simulink model "UAVIntegratedNavigationSystem"  (R2020b)
settings: Solver=FixedStepAuto  StartTime=0.0  StopTime=TFinal  FixedStep=IMUtime  RelTol=1e-3
values from neighbouring files (symbols this model uses):
  AIONtime = 1    [ModelSettings.m]
  BiasAccel = 9.81E-4    (= 0.000981)    [ModelSettings.m]
  BiasGyro = 2.424068405548E-4    (= 0.000242406840555)    [ModelSettings.m]
  CorrTimeOrientationGNSS = 1    [ModelSettings.m]
  CorrTimePositionGNSS = 1    [ModelSettings.m]
  CorrTimeVelocityGNSS = 1    [ModelSettings.m]
  delay = 1.5    [ModelSettings.m]
  e = 0.081819106    [ModelSettings.m]
  g0 = 9.780327    [ModelSettings.m]
  GNSStime = 0.2    [ModelSettings.m]
  H0 = 0.1    [ModelSettings.m]
  IMUtime = 0.01    [ModelSettings.m]
  indUAV = 2    [ModelSettings.m]
  LambdaInit = 0.6555    [ModelSettings.m]
  mass = 0.7    [ModelSettings.m]
  N = 100    [ModelSettings.m]
  PhiInit = 0.968    [ModelSettings.m]
  PitchDown = -PitchUp    (= -0.1)    [ModelSettings.m]
  PitchUp = 0.1    [ModelSettings.m]
  Ra = 6378.245    [ModelSettings.m]
  RollDown = -RollUp    (= -0.1)    [ModelSettings.m]
  RollUp = 0.1    [ModelSettings.m]
  SigmaAccel = 9.81E-4    (= 0.000981)    [ModelSettings.m]
  SigmaAION = 30    [ModelSettings.m]
  SigmaAltitudeGNSS = 3    [ModelSettings.m]
  SigmaGyro = 2.666475246102E-6    (= 2.6664752461e-06)    [ModelSettings.m]
  SigmaLaser = 5    [ModelSettings.m]
  SigmaOrientationGNSS = 0.00349    [ModelSettings.m]
  SigmaPositionGNSS = 1.5    [ModelSettings.m]
  SigmaVelocityGNSS = 0.03    [ModelSettings.m]
  SigmaVelocityUpGNSS = 0.03    [ModelSettings.m]
  U1down = 0    [ModelSettings.m]
  U1up = 4 * ForceCoeff * OmegaMax^2    (= 9.9858124)    [ModelSettings.m]
  U2down = -U2up    (= -2.4964531)    [ModelSettings.m]
  U2up = ForceCoeff * OmegaMax^2    (= 2.4964531)    [ModelSettings.m]
  U3down = -U3up    (= -2.4964531)    [ModelSettings.m]
  U3up = ForceCoeff * OmegaMax^2    (= 2.4964531)    [ModelSettings.m]
  U4down = -U4up    (= -0.2494604)    [ModelSettings.m]
  U4up = 2 * DragCoeff * OmegaMax^2    (= 0.2494604)    [ModelSettings.m]
  WEarth = 7.2921158553E-5    (= 7.2921158553e-05)    [ModelSettings.m]
undefined symbols (not defined in the file or in its folder): deg, Newton, rad, Raphson, s
libraries: simulink x11, sharedtransform x7, pid_lib x6, aerolibconvert2 x4, sharedutil x4
(part 2 of 5)

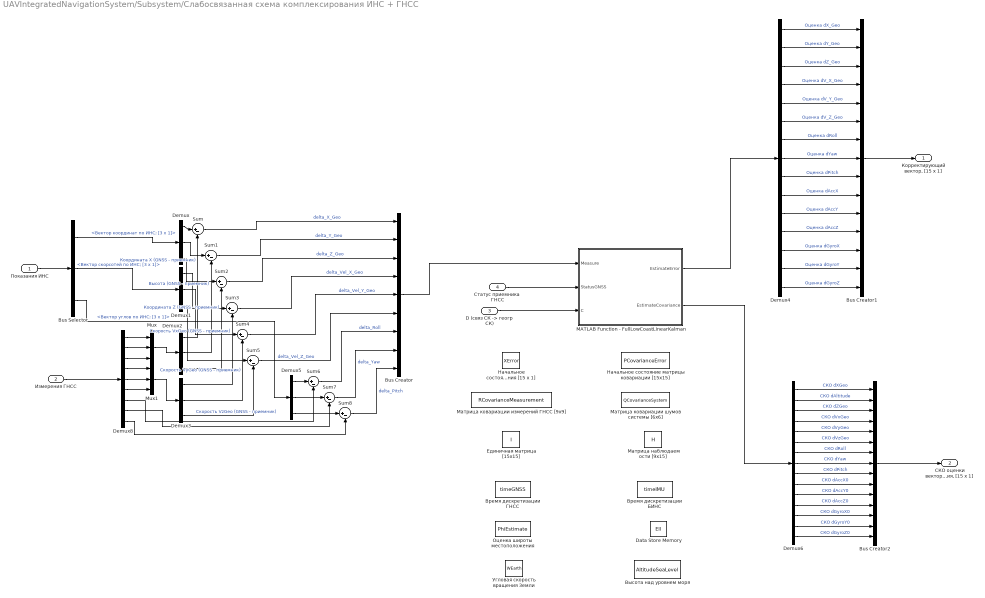
== system UAVIntegratedNavigationSystem/Subsystem/Слабосвязанная схема комплексирования ИНС + ГНСС ==
  Показания ИНС : Inport
  Измерения ГНСС : Inport  Port=2  SampleTime=0.1
  "D (связ СК -> геогр СК)" : Inport  Port=3
  Статус приемника  ГНСС : Inport  Port=4
  Bus Creator : BusCreator  Inputs=9
  Bus Creator1 : BusCreator  Inputs=15
  Bus Creator2 : BusCreator  Inputs=15
  Bus Selector : BusSelector  OutputSignals=Вектор координат по ИНС; [3 x 1],Вектор скорсотей по ИНС; [3 x 1],Вектор углов по ИНС; [3 x 1]
  Data Store Memory : DataStoreMemory  DataStoreName=Ell  ReadBeforeWriteMsg=warning  WriteAfterWriteMsg=warning  WriteAfterReadMsg=warning  InitialValue=[Ra;e]  ShowAdditionalParam=off  OutDataTypeStr=double
  Demux{,1..3,5} (5 alike) : Demux  Outputs=3
  Demux4 : Demux  Outputs=15
  Demux6 : Demux  Outputs=15
  Demux8 : Demux  Outputs=9
  MATLAB Function - FullLowCoastLinearKalman : MATLAB Function  TreatAsAtomicUnit=on
  Mux : Mux  Inputs=3
  Mux1 : Mux  Inputs=3
  Sum{,1..8} (9 alike) : Sum  Inputs=|+-
  Время дискретизации БИНС : DataStoreMemory  DataStoreName=timeIMU  ReadBeforeWriteMsg=warning  WriteAfterWriteMsg=warning  WriteAfterReadMsg=warning  InitialValue=1E-2  ShowAdditionalParam=off  OutDataTypeStr=double
  Время дискретизации ГНСС : DataStoreMemory  DataStoreName=timeGNSS  ReadBeforeWriteMsg=warning  WriteAfterWriteMsg=warning  WriteAfterReadMsg=warning  InitialValue=GNSStime  ShowAdditionalParam=off  OutDataTypeStr=double
  Высота над уровнем моря : DataStoreMemory  DataStoreName=AltitudeSeaLevel  ReadBeforeWriteMsg=warning  WriteAfterWriteMsg=warning  WriteAfterReadMsg=warning  InitialValue=H0  ShowAdditionalParam=off  OutDataTypeStr=double
  Единичная матрица [15x15] : DataStoreMemory  DataStoreName=I  ReadBeforeWriteMsg=warning  WriteAfterWriteMsg=warning  WriteAfterReadMsg=warning  InitialValue=eye(15)  ShowAdditionalParam=off  OutDataTypeStr=double
  Матрица ковариации измерений ГНСС [9x9] : DataStoreMemory  DataStoreName=RCovarianceMeasurement  ReadBeforeWriteMsg=warning  WriteAfterWriteMsg=warning  WriteAfterReadMsg=warning  InitialValue="diag([ (0.1 * SigmaPositionGNSS)^2 (0.1 * SigmaAltitudeGNSS)^2 (0.1 * SigmaPositionGNSS)^2  (1*SigmaVelocityGNSS)^2  (1*SigmaVelocityUpGNSS)^2 (1*SigmaVelocityGNSS)^2 (0.001*SigmaOrientationGNSS)^2 (0.001*SigmaOrientationGNSS)^2 (0.001*SigmaOrientationGNSS)^2])"  ShowAdditionalParam=off  OutDataTypeStr=double
  Матрица ковариации шумов системы [6x6] : DataStoreMemory  DataStoreName=QCovarianceSystem  ReadBeforeWriteMsg=warning  WriteAfterWriteMsg=warning  WriteAfterReadMsg=warning  InitialValue=diag([SigmaAccel^2 SigmaAccel^2 SigmaAccel^2 SigmaGyro^2 SigmaGyro^2 SigmaGyro^2])  ShowAdditionalParam=off  OutDataTypeStr=double
  Матрица наблюдаемости [9x15] : DataStoreMemory  DataStoreName=H  ReadBeforeWriteMsg=warning  WriteAfterWriteMsg=warning  WriteAfterReadMsg=warning  InitialValue=[1 0 0 0 0 0 0 0 0 0 0 0 0 0 0;0 1 0 0 0 0 0 0 0 0 0 0 0 0 0; 0 0 1 0 0 0 0 0 0 0 0 0 0 0 0; 0 0 0 1 0 0 0 0 0 0 0 0 0 0 0; 0 0 0 0 1 0 0 0 0 0 0 0 0 0 0; 0 0 0 0 0 1 0 0 0 0 0 0 0 0 0; 0 0 0 0 0 0 1 0 0 0 0 0 0 0 0; 0 0 0 0 0 0 0 1 0 0 0 0 0 0 0; 0 0 0 0 0 0 0 0 1 0 0 0 0 0 0]  ShowAdditionalParam=off  OutDataTypeStr=double
  Начальное состояние вектора - состояния [15 x 1] : DataStoreMemory  DataStoreName=XError  ReadBeforeWriteMsg=warning  WriteAfterWriteMsg=warning  WriteAfterReadMsg=warning  InitialValue=[0;0;0;0;0;0;0;0;0;0;0;0;0;0;0]  ShowAdditionalParam=off  OutDataTypeStr=double
  Начальное состояние матрицы ковариации [15x15] : DataStoreMemory  DataStoreName=PCovarianceError  ReadBeforeWriteMsg=warning  WriteAfterWriteMsg=warning  WriteAfterReadMsg=warning  InitialValue=diag([10 10 10 2 2 2 1e-1 1e-1 1e-1 1e-3 1e-3 1e-3 1e-3 1e-3 1e-3])  ShowAdditionalParam=off  OutDataTypeStr=double
  Оценка широты местоположения : DataStoreMemory  DataStoreName=PhiEstimate  ReadBeforeWriteMsg=warning  WriteAfterWriteMsg=warning  WriteAfterReadMsg=warning  InitialValue=PhiInit  ShowAdditionalParam=off  OutDataTypeStr=double
  Угловая скорость вращения Земли : DataStoreMemory  DataStoreName=WEarth  ReadBeforeWriteMsg=warning  WriteAfterWriteMsg=warning  WriteAfterReadMsg=warning  InitialValue=WEarth  ShowAdditionalParam=off  OutDataTypeStr=double
  "Корректирующий вектор, [15 x 1]" : Outport
  "СКО оценки вектора состояния, [15 x 1]" : Outport  Port=2
  wires:
  Показания ИНС/1 -> Bus Selector/1
  Sum/1 -> Bus Creator/1  "delta_X_Geo"
  Sum1/1 -> Bus Creator/2  "delta_Y_Geo"
  Sum2/1 -> Bus Creator/3  "delta_Z_Geo"
  Sum3/1 -> Bus Creator/4  "delta_Vel_X_Geo"
  Sum4/1 -> Bus Creator/5  "delta_Vel_Y_Geo"
  Demux3/2 -> Sum4/2  "Скорость VyGeo (GNSS - приемник)"
  Sum5/1 -> Bus Creator/6  "delta_Vel_Z_Geo"
  Demux3/3 -> Sum5/2  "Скорость VzGeo (GNSS - приемник)"
  Bus Selector/1 -> Demux/1  "<Вектор координат по ИНС; [3 x 1]>"
  Bus Selector/2 -> Demux1/1  "<Вектор скорсотей по ИНС; [3 x 1]>"
  Demux8/1 -> Mux/1
  Demux8/2 -> Mux/2
  Demux8/3 -> Mux/3
  Mux/1 -> Demux2/1
  Demux8/4 -> Mux1/1
  Demux8/5 -> Mux1/2
  Demux8/6 -> Mux1/3
  Mux1/1 -> Demux3/1
  Demux6/1 -> Bus Creator2/1  "СКО dXGeo"
  Demux6/2 -> Bus Creator2/2  "СКО dAltitude"
  Demux6/3 -> Bus Creator2/3  "СКО dZGeo"
  Demux6/4 -> Bus Creator2/4  "СКО dVxGeo"
  Demux6/5 -> Bus Creator2/5  "СКО dVyGeo"
  Demux6/6 -> Bus Creator2/6  "СКО dVzGeo"
  Demux/1 -> Sum/1
  Demux2/1 -> Sum/2  "Координата X (GNSS - приемник)"
  Demux/2 -> Sum1/1
  Demux2/2 -> Sum1/2  "Высота (GNSS - приемник)"
  Demux2/3 -> Sum2/2  "Координата Z (GNSS - приемник)"
  Demux/3 -> Sum2/1
  Demux1/1 -> Sum3/1
  Demux3/1 -> Sum3/2  "Скорость VxGeo (GNSS - приемник)"
  Demux1/3 -> Sum5/1
  Demux1/2 -> Sum4/1
  Demux4/1 -> Bus Creator1/1  "Оценка dX_Geo"
  Demux4/2 -> Bus Creator1/2  "Оценка dY_Geo"
  Demux4/3 -> Bus Creator1/3  "Оценка dZ_Geo"
  Demux4/4 -> Bus Creator1/4  "Оценка dV_X_Geo"
  Demux4/5 -> Bus Creator1/5  "Оценка dV_Y_Geo"
  Demux4/6 -> Bus Creator1/6  "Оценка dV_Z_Geo"
  Demux4/7 -> Bus Creator1/7  "Оценка dRoll"
  Demux4/8 -> Bus Creator1/8  "Оценка dYaw"
  Demux4/9 -> Bus Creator1/9  "Оценка dPitch"
  Demux6/7 -> Bus Creator2/7  "СКО dRoll"
  Demux6/8 -> Bus Creator2/8  "СКО dYaw"
  Demux6/9 -> Bus Creator2/9  "СКО dPitch"
  Bus Creator2/1 -> "СКО оценки вектора состояния, [15 x 1]"/1
  "D (связ СК -> геогр СК)"/1 -> MATLAB Function - FullLowCoastLinearKalman/3(C)
  Bus Selector/3 -> Demux5/1  "<Вектор углов по ИНС; [3 x 1]>"
  Demux5/1 -> Sum6/1
  Demux8/7 -> Sum6/2
  Sum6/1 -> Bus Creator/7  "delta_Roll"
  Demux5/2 -> Sum7/1
  Sum7/1 -> Bus Creator/8  "delta_Yaw"
  Demux8/8 -> Sum7/2
  Demux5/3 -> Sum8/1
  Sum8/1 -> Bus Creator/9  "delta_Pitch"
  Demux8/9 -> Sum8/2
  Bus Creator/1 -> MATLAB Function - FullLowCoastLinearKalman/1(Measure)
  Demux6/10 -> Bus Creator2/10  "СКО dAccX0"
  Demux6/11 -> Bus Creator2/11  "СКО dAccY0"
  Demux6/12 -> Bus Creator2/12  "СКО dAccZ0"
  Demux6/13 -> Bus Creator2/13  "СКО dGyroX0"
  Demux6/14 -> Bus Creator2/14  "СКО dGyroY0"
  Demux6/15 -> Bus Creator2/15  "СКО dGyroZ0"
  Demux4/10 -> Bus Creator1/10  "Оценка dAccX"
  Demux4/11 -> Bus Creator1/11  "Оценка dAccY"
  Demux4/12 -> Bus Creator1/12  "Оценка dAccZ"
  Demux4/13 -> Bus Creator1/13  "Оценка dGyroX"
  Demux4/14 -> Bus Creator1/14  "Оценка dGyroY"
  Demux4/15 -> Bus Creator1/15  "Оценка dGyroZ"
  MATLAB Function - FullLowCoastLinearKalman/2(EstimateCovariance) -> Demux6/1
  Измерения ГНСС/1 -> Demux8/1
  Статус приемника  ГНСС/1 -> MATLAB Function - FullLowCoastLinearKalman/2(StatusGNSS)
  MATLAB Function - FullLowCoastLinearKalman/1(EstimateError) -> Demux4/1
  Bus Creator1/1 -> "Корректирующий вектор, [15 x 1]"/1

== system UAVIntegratedNavigationSystem/Subsystem1/Функционирование АИОН ==
  КОИ : Inport
  Измерения АИОН : Inport  Port=2
  Bus Creator : BusCreator  Inputs=3
  Data Store Memory : DataStoreMemory  DataStoreName=sum  ReadBeforeWriteMsg=warning  WriteAfterWriteMsg=warning  WriteAfterReadMsg=warning  ShowAdditionalParam=off  OutDataTypeStr=double
  Demux : Demux  Outputs=3
  If Action Subsystem1 : Subsystem  TreatAsAtomicUnit=on
  If Action Subsystem3 : Subsystem  TreatAsAtomicUnit=on
  If Action Subsystem4 : Subsystem  TreatAsAtomicUnit=on
  If Action Subsystem5 : Subsystem  TreatAsAtomicUnit=on
  MATLAB Function : MATLAB Function  TreatAsAtomicUnit=on
  Merge : Merge
  Merge1 : Merge
  Rate Transition : RateTransition  OutPortSampleTime=AIONtime
  Моменты получения информации с АИОН : DiscretePulseGenerator  PulseType=Time based  Period=AIONtime  PulseWidth=10  PhaseDelay=GNSStime
  Отказ  АИОН : If  IfExpression=u1 == 2
  Пропадание имзерений АИОН : If  IfExpression=u1 == -1
  Измерения АИОН (выход) : Outport
  Статус АИОН (-1/0 / 1) : Outport  Port=2
  Количество отсчетов после проадания сигнала АИОН : Outport  Port=3
  wires:
  If Action Subsystem1/1(Out1) -> Merge/1
  If Action Subsystem3/1(Out1) -> Merge/2
  Пропадание имзерений АИОН/1 -> If Action Subsystem4/Action
  Измерения АИОН/1 -> If Action Subsystem5/1(In1)
  Пропадание имзерений АИОН/2 -> If Action Subsystem5/Action
  If Action Subsystem4/1(Out1) -> Merge1/1
  If Action Subsystem5/1(Out1) -> Merge1/2
  Merge1/1 -> Demux/1
  КОИ/1 -> Отказ  АИОН/1
  Отказ  АИОН/1 -> If Action Subsystem1/Action
  Отказ  АИОН/2 -> If Action Subsystem3/Action
  Моменты получения информации с АИОН/1 -> If Action Subsystem1/1(In1)
  Demux/1 -> Bus Creator/1  "X_Geo_AION"
  Demux/2 -> Bus Creator/2  "Altitude_AION"
  Demux/3 -> Bus Creator/3  "Z_Geo_AION"
  Bus Creator/1 -> Измерения АИОН (выход)/1
  Merge/1 -> Статус АИОН (-1/0 / 1)/1, MATLAB Function/1(AIONStatus), Пропадание имзерений АИОН/1
  MATLAB Function/1(y) -> Rate Transition/1
  Rate Transition/1 -> Количество отсчетов после проадания сигнала АИОН/1

== system UAVIntegratedNavigationSystem/Subsystem1/Функционирование приемника ГНСС ==
  КОИ : Inport
  Измерения приемника ГНСС : Inport  Port=2
  Bus Creator : BusCreator  Inputs=3
  Data Store Memory : DataStoreMemory  DataStoreName=sum  ReadBeforeWriteMsg=warning  WriteAfterWriteMsg=warning  WriteAfterReadMsg=warning  ShowAdditionalParam=off  OutDataTypeStr=double
  Demux : Demux  Outputs=9
  If Action Subsystem1 : Subsystem  TreatAsAtomicUnit=on
  If Action Subsystem3 : Subsystem  TreatAsAtomicUnit=on
  If Action Subsystem4 : Subsystem  TreatAsAtomicUnit=on
  If Action Subsystem5 : Subsystem  TreatAsAtomicUnit=on
  MATLAB Function : MATLAB Function  TreatAsAtomicUnit=on
  Merge : Merge
  Merge1 : Merge
  Mux : Mux  Inputs=3
  Mux1 : Mux  Inputs=3
  Mux2 : Mux  Inputs=3
  Rate Transition : RateTransition  OutPortSampleTime=GNSStime
  Моменты получения информации с ГНСС : DiscretePulseGenerator  PulseType=Time based  Period=GNSStime  PulseWidth=10  PhaseDelay=GNSStime
  Отказ  приемника ГНСС : If  IfExpression=u1 == 1
  Пропадание измерений приемника ГНСС : If  IfExpression=u1 == -1
  Измерения приемника ГНСС (выход) : Outport
  Статус приемника (-1/0 / 1) : Outport  Port=2
  Количество отсчетов после проадания сигнала ГНСС : Outport  Port=3
  wires:
  If Action Subsystem1/1(Out1) -> Merge/1
  If Action Subsystem3/1(Out1) -> Merge/2
  Пропадание измерений приемника ГНСС/1 -> If Action Subsystem4/Action
  Измерения приемника ГНСС/1 -> If Action Subsystem5/1(In1)
  Пропадание измерений приемника ГНСС/2 -> If Action Subsystem5/Action
  If Action Subsystem4/1(Out1) -> Merge1/1
  If Action Subsystem5/1(Out1) -> Merge1/2
  КОИ/1 -> Отказ  приемника ГНСС/1
  Отказ  приемника ГНСС/1 -> If Action Subsystem1/Action
  Отказ  приемника ГНСС/2 -> If Action Subsystem3/Action
  Merge/1 -> Статус приемника (-1/0 / 1)/1, Пропадание измерений приемника ГНСС/1, MATLAB Function/1(GNSSStatus)
  Моменты получения информации с ГНСС/1 -> If Action Subsystem1/1(In1)
  Merge1/1 -> Demux/1
  Demux/1 -> Mux/1
  Demux/2 -> Mux/2
  Demux/3 -> Mux/3
  Mux/1 -> Bus Creator/1  "Вектор координат по ГНСС; [3 x 1]"
  Demux/4 -> Mux1/1
  Demux/5 -> Mux1/2
  Demux/6 -> Mux1/3
  Mux1/1 -> Bus Creator/2  "Вектор скоростей по ГНСС; [3 x 1]"
  Bus Creator/1 -> Измерения приемника ГНСС (выход)/1
  Demux/8 -> Mux2/2
  Demux/9 -> Mux2/3
  Demux/7 -> Mux2/1
  Mux2/1 -> Bus Creator/3  "Вектор углов по ГНСС; [3 x 1]"
  MATLAB Function/1(y) -> Rate Transition/1
  Rate Transition/1 -> Количество отсчетов после проадания сигнала ГНСС/1

== system UAVIntegratedNavigationSystem/Алгоритм ИНС /Алгоритм Навигации ==
  Показания акселерометров (геогр СК) : Inport
  "Север(0), Восток(0)" : Inport  Port=2
  Demux : Demux  Outputs=3
  Demux1 : Demux
  Mux : Mux  Inputs=3
  Mux1 : Mux  Inputs=2
  Координаты БПЛА (Географ. СК) : Subsystem
  Радиус - вектор точки местоположения Ц.М. БПЛА (phi) : Subsystem
  Скорости БПЛА (Географ. СК) : Subsystem
  Угловая скорость вращения трехгранника : Subsystem
  "Координаты, скорости БЛА" : Outport
  OmegaG : Outport  Port=2
  Широта местоположения БЛА : Outport  Port=3
  "Радиусы кривизны земного эллипсоида, м" : Outport  Port=4
  wires:
  Demux/1 -> Скорости БПЛА (Географ. СК)/1(AccX)  "AccX"
  Demux/2 -> Скорости БПЛА (Географ. СК)/2(AccY)  "AccY"
  Demux/3 -> Скорости БПЛА (Географ. СК)/3(AccZ)  "AccZ"
  Показания акселерометров (геогр СК)/1 -> Demux/1
  Координаты БПЛА (Географ. СК)/1("Coord, phi") -> Demux1/1
  Demux1/4 -> Угловая скорость вращения трехгранника/3(phi), Скорости БПЛА (Географ. СК)/5(phi), Радиус - вектор точки местоположения Ц.М. БПЛА (phi)/1(Phi), Широта местоположения БЛА/1
  Радиус - вектор точки местоположения Ц.М. БПЛА (phi)/1("R, м") -> Скорости БПЛА (Географ. СК)/4(R), Угловая скорость вращения трехгранника/2(R), Координаты БПЛА (Географ. СК)/2(R), "Радиусы кривизны земного эллипсоида, м"/1
  Угловая скорость вращения трехгранника/1(OmegaG) -> OmegaG/1
  Demux1/1 -> Mux/1
  Demux1/2 -> Mux/2
  Demux1/3 -> Mux/3
  Mux1/1 -> "Координаты, скорости БЛА"/1
  Скорости БПЛА (Географ. СК)/1(Velocity) -> Mux1/2, Угловая скорость вращения трехгранника/1(Velocity), Координаты БПЛА (Географ. СК)/1(Velocity)
  Mux/1 -> Mux1/1
  "Север(0), Восток(0)"/1 -> Координаты БПЛА (Географ. СК)/3("Север(0), Восток(0)")

== system UAVIntegratedNavigationSystem/Алгоритм ИНС /Алгоритм Ориентации ==
  Показания ДУС (связ СК) : Inport
  OmegaG : Inport  Port=2
  Add : Sum  Inputs=-+
  Demux : Demux  Outputs=3
  Integrator : Integrator  InitialCondition=[1, 0, 0, 0]
  Matrix Multiply : Product  Multiplication=Matrix(*)
  Mux : Mux  Inputs=3
  Mux4 : Mux  Inputs=2
  Quaternions to Rotation Angles : sharedtransform/Quaternions to Rotation Angles  rotationOrder=YZX  aMode=aMode
      settings: SourceProductBaseCode=AE,PW,MT,UV,VE,VP
  Rotation Angles to Direction Cosine Matrix : sharedtransform/Rotation Angles to Direction Cosine Matrix  rotationOrder=YZX  aMode=aMode
      settings: SourceProductBaseCode=AE,PW,MT,UV,VE,VP
  ДУ кватерниона : Subsystem
  Нормирование кватерниона : Subsystem
  "Матрица перевода D(связ СК -> геогр СК)" : Outport
  wires:
  ДУ кватерниона/1(d(Q)/dt) -> Integrator/1
  Quaternions to Rotation Angles/1 -> Rotation Angles to Direction Cosine Matrix/1
  Integrator/1 -> Нормирование кватерниона/1(q)
  Нормирование кватерниона/1(qnorm) -> Mux4/2, Quaternions to Rotation Angles/1
  Mux4/1 -> ДУ кватерниона/1(state)  "Wx Wz Wy  Q0-Q3"
  Mux/1 -> Add/2
  Demux/1 -> Mux/1  "AngX"
  Demux/2 -> Mux/2  "AngY"
  Demux/3 -> Mux/3  "AngZ"
  Показания ДУС (связ СК)/1 -> Demux/1
  Rotation Angles to Direction Cosine Matrix/1 -> Matrix Multiply/1, "Матрица перевода D(связ СК -> геогр СК)"/1
  Add/1 -> Mux4/1
  Matrix Multiply/1 -> Add/1
  OmegaG/1 -> Matrix Multiply/2

== system UAVIntegratedNavigationSystem/Алгоритм ИНС /Блок ошибок ДУС ==
  Истинные значения : Inport
  Add : Sum  Inputs=+++
  Band-Limited White Noise1 : simulink/Sources/Band-Limited White Noise  Cov=[IMUtime]  Ts=IMUtime  seed=[23341]
  BiasGyro : Constant  Value=BiasGyro
  Mux1 : Mux  Inputs=3
  Mux4 : Mux  Inputs=3
  sigma : Gain  Gain=SigmaGyro
  Показания ДУС : Outport
  wires:
  Mux4/1 -> Add/1
  BiasGyro/1 -> Mux4/3, Mux4/2, Mux4/1
  Add/1 -> Показания ДУС/1
  Истинные значения/1 -> Add/2
  Mux1/1 -> Add/3
  Band-Limited White Noise1/1 -> sigma/1
  sigma/1 -> Mux1/1, Mux1/3, Mux1/2

== system UAVIntegratedNavigationSystem/Алгоритм ИНС /Блок ошибок акселерометров ==
  Истинные значения : Inport
  Add1 : Sum  Inputs=+++
  Band-Limited White Noise1 : simulink/Sources/Band-Limited White Noise  Cov=[IMUtime]  Ts=IMUtime  seed=[23341]
  BiasAccel : Constant  Value=BiasAccel
  Mux1 : Mux  Inputs=3
  Mux5 : Mux  Inputs=3
  sigma : Gain  Gain=SigmaAccel
  Показания акселерометров : Outport
  wires:
  BiasAccel/1 -> Mux5/3, Mux5/2, Mux5/1
  Add1/1 -> Показания акселерометров/1
  Истинные значения/1 -> Add1/2
  Mux5/1 -> Add1/1
  sigma/1 -> Mux1/1, Mux1/3, Mux1/2
  Band-Limited White Noise1/1 -> sigma/1
  Mux1/1 -> Add1/3

== system UAVIntegratedNavigationSystem/Алгоритм ИНС /Блок пересчета ==
  "D (связ СК -> геогр СК)" : Inport
  Показания акселерометров (связ СК) : Inport  Port=2
  Matrix Multiply : Product  Multiplication=Matrix(*)
  Показания акселерометров (геогр СК) : Outport
  wires:
  Показания акселерометров (связ СК)/1 -> Matrix Multiply/2
  "D (связ СК -> геогр СК)"/1 -> Matrix Multiply/1
  Matrix Multiply/1 -> Показания акселерометров (геогр СК)/1

== system UAVIntegratedNavigationSystem/Алгоритм ИНС /Вычисление углов ==
  "D (связ СК -> геогр СК)" : Inport
  Demux : Demux  Outputs=3
  Direction Cosine Matrix to Rotation Angles : sharedtransform/Direction Cosine Matrix to Rotation Angles  rotationOrder=YZX  aMode=aMode  action=None  tolerance=eps(2)
      settings: SourceProductBaseCode=AE,PW,MT,UV,VE,VP
  Mux : Mux  Inputs=3
  Углы ориентации : Outport
  wires:
  Direction Cosine Matrix to Rotation Angles/1 -> Demux/1
  "D (связ СК -> геогр СК)"/1 -> Direction Cosine Matrix to Rotation Angles/1
  Demux/1 -> Mux/2  "Psi"
  Demux/2 -> Mux/3  "Pitch"
  Demux/3 -> Mux/1  "Roll"
  Mux/1 -> Углы ориентации/1

== system UAVIntegratedNavigationSystem/Алгоритм ИНС (коррекия БЧЭ)/Алгоритм Навигации ==
  Показания акселерометров (геогр СК) : Inport
  "Север(0), Восток(0)" : Inport  Port=2
  Demux : Demux  Outputs=3
  Demux1 : Demux
  Mux : Mux  Inputs=3
  Mux1 : Mux  Inputs=2
  Координаты БПЛА (Географ. СК) : Subsystem
  Радиус - вектор точки местоположения Ц.М. БПЛА (phi) : Subsystem
  Скорости БПЛА (Географ. СК) : Subsystem
  Угловая скорость вращения трехгранника : Subsystem
  "Координаты, скорости БЛА" : Outport
  OmegaG : Outport  Port=2
  wires:
  Demux/1 -> Скорости БПЛА (Географ. СК)/1(AccX)  "AccX"
  Demux/2 -> Скорости БПЛА (Географ. СК)/2(AccY)  "AccY"
  Demux/3 -> Скорости БПЛА (Географ. СК)/3(AccZ)  "AccZ"
  Показания акселерометров (геогр СК)/1 -> Demux/1
  Координаты БПЛА (Географ. СК)/1("Coord, phi") -> Demux1/1
  Demux1/4 -> Угловая скорость вращения трехгранника/3(phi), Скорости БПЛА (Географ. СК)/5(phi), Радиус - вектор точки местоположения Ц.М. БПЛА (phi)/1(Phi)
  Радиус - вектор точки местоположения Ц.М. БПЛА (phi)/1("R, м") -> Скорости БПЛА (Географ. СК)/4(R), Угловая скорость вращения трехгранника/2(R), Координаты БПЛА (Географ. СК)/2(R)
  Угловая скорость вращения трехгранника/1(OmegaG) -> OmegaG/1
  Demux1/1 -> Mux/1
  Demux1/2 -> Mux/2
  Demux1/3 -> Mux/3
  Mux1/1 -> "Координаты, скорости БЛА"/1
  Скорости БПЛА (Географ. СК)/1(Velocity) -> Mux1/2, Угловая скорость вращения трехгранника/1(Velocity), Координаты БПЛА (Географ. СК)/1(Velocity)
  Mux/1 -> Mux1/1
  "Север(0), Восток(0)"/1 -> Координаты БПЛА (Географ. СК)/3("Север(0), Восток(0)")

== system UAVIntegratedNavigationSystem/Алгоритм ИНС (коррекия БЧЭ)/Алгоритм Ориентации ==
  Показания ДУС (связ СК) : Inport
  OmegaG : Inport  Port=2
  Add : Sum  Inputs=-+
  Demux : Demux  Outputs=3
  Integrator : Integrator  InitialCondition=[1, 0, 0, 0]
  Matrix Multiply : Product  Multiplication=Matrix(*)
  Mux : Mux  Inputs=3
  Mux4 : Mux  Inputs=2
  Quaternions to Rotation Angles : sharedtransform/Quaternions to Rotation Angles  rotationOrder=YZX  aMode=aMode
      settings: SourceProductBaseCode=AE,PW,MT,UV,VE,VP
  Rotation Angles to Direction Cosine Matrix : sharedtransform/Rotation Angles to Direction Cosine Matrix  rotationOrder=YZX  aMode=aMode
      settings: SourceProductBaseCode=AE,PW,MT,UV,VE,VP
  ДУ кватерниона : Subsystem
  Нормирование кватерниона : Subsystem
  "Матрица перевода D(связ СК -> геогр СК)" : Outport
  wires:
  ДУ кватерниона/1(d(Q)/dt) -> Integrator/1
  Quaternions to Rotation Angles/1 -> Rotation Angles to Direction Cosine Matrix/1
  Integrator/1 -> Нормирование кватерниона/1(q)
  Нормирование кватерниона/1(qnorm) -> Mux4/2, Quaternions to Rotation Angles/1
  Mux4/1 -> ДУ кватерниона/1(state)  "Wx Wz Wy  Q0-Q3"
  Mux/1 -> Add/2
  Demux/1 -> Mux/1  "AngX"
  Demux/2 -> Mux/2  "AngY"
  Demux/3 -> Mux/3  "AngZ"
  Показания ДУС (связ СК)/1 -> Demux/1
  Rotation Angles to Direction Cosine Matrix/1 -> Matrix Multiply/1, "Матрица перевода D(связ СК -> геогр СК)"/1
  Add/1 -> Mux4/1
  Matrix Multiply/1 -> Add/1
  OmegaG/1 -> Matrix Multiply/2

== system UAVIntegratedNavigationSystem/Алгоритм ИНС (коррекия БЧЭ)/Блок ошибок ДУС ==
  Истинные значения : Inport
  +-1000 град/сек : Saturate  UpperLimit=17.45  LowerLimit=-17.45
  Add : Sum  Inputs=+++
  Angular Velocity Conversion : aerolibconvert2/Angular Velocity Conversion  IU=rad/s  OU=deg/s
  Band-Limited White Noise1 : simulink/Sources/Band-Limited White Noise  Cov=[IMUtime]  Ts=IMUtime  seed=[23341]
  BiasGyro : Constant  Value=BiasGyro
  Demux : Demux  Outputs=3
  Mux1 : Mux  Inputs=3
  Mux4 : Mux  Inputs=3
  To Workspace : ToWorkspace  VariableName=AngleVelBF_X  SaveFormat=Timeseries  SampleTime=IMUtime
  To Workspace1 : ToWorkspace  VariableName=AngleVelBF_Y  SaveFormat=Timeseries  SampleTime=IMUtime
  To Workspace2 : ToWorkspace  VariableName=AngleVelBF_Z  SaveFormat=Timeseries  SampleTime=IMUtime
  sigma : Gain  Gain=SigmaGyro
  Показания ДУС : Outport
  wires:
  Mux4/1 -> Add/1
  BiasGyro/1 -> Mux4/3, Mux4/2, Mux4/1
  Add/1 -> +-1000 град/сек/1
  Истинные значения/1 -> Add/2
  Mux1/1 -> Add/3
  Band-Limited White Noise1/1 -> sigma/1
  sigma/1 -> Mux1/1, Mux1/3, Mux1/2
  Angular Velocity Conversion/1 -> Demux/1
  Demux/1 -> To Workspace/1  "AngleVelBF_X"
  Demux/2 -> To Workspace1/1  "AngleVelBF_Y"
  Demux/3 -> To Workspace2/1  "AngleVelBF_Z"
  +-1000 град/сек/1 -> Показания ДУС/1, Angular Velocity Conversion/1

== system UAVIntegratedNavigationSystem/Алгоритм ИНС (коррекия БЧЭ)/Блок ошибок акселерометров ==
  Истинные значения : Inport
  +-10g : Saturate  UpperLimit=10 * g0  LowerLimit=-10 * g0
  Add1 : Sum  Inputs=+++
  Band-Limited White Noise1 : simulink/Sources/Band-Limited White Noise  Cov=[IMUtime]  Ts=IMUtime  seed=[23341]
  BiasAccel : Constant  Value=BiasAccel
  Mux1 : Mux  Inputs=3
  Mux5 : Mux  Inputs=3
  sigma : Gain  Gain=SigmaAccel
  Показания акселерометров : Outport
  wires:
  BiasAccel/1 -> Mux5/3, Mux5/2, Mux5/1
  Add1/1 -> +-10g/1
  Истинные значения/1 -> Add1/2
  Mux5/1 -> Add1/1
  sigma/1 -> Mux1/1, Mux1/3, Mux1/2
  Band-Limited White Noise1/1 -> sigma/1
  Mux1/1 -> Add1/3
  +-10g/1 -> Показания акселерометров/1

== system UAVIntegratedNavigationSystem/Алгоритм ИНС (коррекия БЧЭ)/Блок пересчета ==
  "D (связ СК -> геогр СК)" : Inport
  Показания акселерометров (связ СК) : Inport  Port=2
  Matrix Multiply : Product  Multiplication=Matrix(*)
  Показания акселерометров (геогр СК) : Outport
  wires:
  Показания акселерометров (связ СК)/1 -> Matrix Multiply/2
  "D (связ СК -> геогр СК)"/1 -> Matrix Multiply/1
  Matrix Multiply/1 -> Показания акселерометров (геогр СК)/1

== system UAVIntegratedNavigationSystem/Алгоритм ИНС (коррекия БЧЭ)/Вычисление углов ==
  "D (связ СК -> геогр СК)" : Inport
  Demux : Demux  Outputs=3
  Direction Cosine Matrix to Rotation Angles : sharedtransform/Direction Cosine Matrix to Rotation Angles  rotationOrder=YZX  aMode=aMode  action=None  tolerance=eps(2)
      settings: SourceProductBaseCode=AE,PW,MT,UV,VE,VP
  Mux : Mux  Inputs=3
  Углы ориентации : Outport
  wires:
  Direction Cosine Matrix to Rotation Angles/1 -> Demux/1
  "D (связ СК -> геогр СК)"/1 -> Direction Cosine Matrix to Rotation Angles/1
  Demux/1 -> Mux/2  "Psi"
  Demux/2 -> Mux/3  "Pitch"
  Demux/3 -> Mux/1  "Roll"
  Mux/1 -> Углы ориентации/1

== system UAVIntegratedNavigationSystem/Блок модели динамики квадрокоптера + САУ/Полетный контроллер ==
  Высота заданная : Inport
  "  Z заданная" : Inport  Port=2
  X заданная : Inport  Port=3
  Курс заданный : Inport  Port=4
  <Y> : Inport  Port=5
  <Z> : Inport  Port=6
  <X> : Inport  Port=7
  <Roll> : Inport  Port=8
  <Psi> : Inport  Port=9
  <Pitch> : Inport  Port=10
  g : Inport  Port=11
  Параметры САУ БпЛА : Inport  Port=12
  Bus Selector : BusSelector  OutputSignals=AltPID,ZPID,XPID,RollPID,PitchPID,PsiPID
  Ограничение (-pi / pi) : Saturate  UpperLimit=pi  LowerLimit=-pi
  Ограничение управляющих сил : Subsystem
  Угловая стабилизация : Subsystem
  "Удержание высоты " : Subsystem
  Удержание положения : Subsystem
  U1 : Outport
  U2 : Outport  Port=2
  U3 : Outport  Port=3
  U4 : Outport  Port=4
  wires:
  Удержание положения/2(Pitch*) -> Угловая стабилизация/3(Pitch*)
  Угловая стабилизация/3(U4*) -> Ограничение управляющих сил/4(U4*)
  "Удержание высоты "/1(U1*) -> Ограничение управляющих сил/1(U1*)
  Угловая стабилизация/2(U3*) -> Ограничение управляющих сил/3(U3*)
  Ограничение управляющих сил/1(U1) -> Удержание положения/5(U1), U1/1
  Удержание положения/1(Roll*) -> Угловая стабилизация/1(Roll*)
  X заданная/1 -> Удержание положения/3(X*)
  Курс заданный/1 -> Ограничение (-pi / pi)/1
  Угловая стабилизация/1(U2*) -> Ограничение управляющих сил/2(U2*)
  <Z>/1 -> Удержание положения/2(Z)
  Ограничение управляющих сил/2(U2) -> U2/1
  Ограничение управляющих сил/4(U4) -> U4/1
  Ограничение управляющих сил/3(U3) -> U3/1
  <X>/1 -> Удержание положения/4(X)
  <Roll>/1 -> Угловая стабилизация/2(Roll)
  <Pitch>/1 -> Угловая стабилизация/4(Pitch)
  <Psi>/1 -> Удержание положения/6(Psi), Угловая стабилизация/6(Psi)
  Ограничение (-pi / pi)/1 -> Угловая стабилизация/5(Psi*)
  Высота заданная/1 -> "Удержание высоты "/1(Y*)
  "  Z заданная"/1 -> Удержание положения/1(Z*)
  <Y>/1 -> "Удержание высоты "/2(Y)
  g/1 -> "Удержание высоты "/3(g)
  Параметры САУ БпЛА/1 -> Bus Selector/1
  Bus Selector/1 -> "Удержание высоты "/4(AltPID)  "<AltPID>"
  Bus Selector/2 -> Удержание положения/7(ZPID)  "<ZPID>"
  Bus Selector/3 -> Удержание положения/8(XPID)  "<XPID>"
  Bus Selector/4 -> Угловая стабилизация/7(RollPID)  "<RollPID>"
  Bus Selector/5 -> Угловая стабилизация/8(PitchPID)  "<PitchPID>"
  Bus Selector/6 -> Угловая стабилизация/9(PsiPID)  "<PsiPID>"

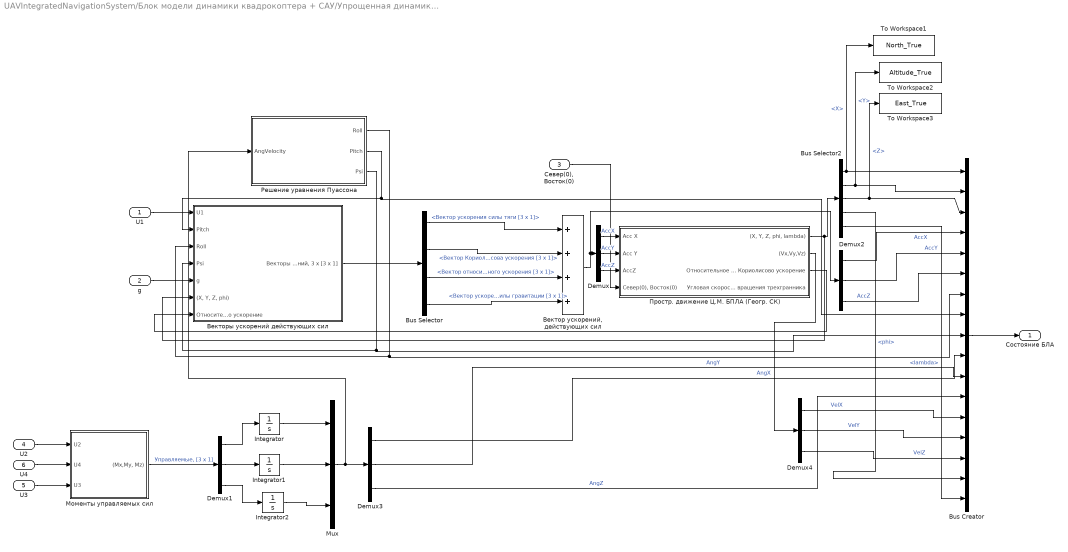
== system UAVIntegratedNavigationSystem/Блок модели динамики квадрокоптера + САУ/Упрощенная динамика БЛА  ==
  U1 : Inport
  g : Inport  Port=2
  "Север(0), Восток(0)" : Inport  Port=3
  U2 : Inport  Port=4
  U3 : Inport  Port=5
  U4 : Inport  Port=6
  Bus Creator : BusCreator  Inputs=17
  Bus Selector : BusSelector  OutputSignals=Вектор ускорения силы тяги [3 x 1],Вектор Кориолисова ускорения [3 x 1],Вектор относительного ускорения [3 x 1],Вектор ускорения силы гравитации [3 x 1]
  Bus Selector2 : BusSelector  OutputSignals=X,Y,Z,phi,lambda
  Demux{,1..4} (5 alike) : Demux  Outputs=3
  Integrator : Integrator
  Integrator1 : Integrator
  Integrator2 : Integrator
  Mux : Mux  Inputs=3
  To Workspace1 : ToWorkspace  VariableName=North_True  SaveFormat=Timeseries  SampleTime=IMUtime
  To Workspace2 : ToWorkspace  VariableName=Altitude_True  SaveFormat=Timeseries  SampleTime=IMUtime
  To Workspace3 : ToWorkspace  VariableName=East_True  SaveFormat=Timeseries  SampleTime=IMUtime
  "Вектор ускорений, действующих сил" : Sum  Inputs=++++
  Векторы ускорений действующих сил : Subsystem
  Моменты управляемых сил : Subsystem
  Простр. движение Ц.М. БПЛА (Геогр. СК) : Subsystem
  Решение уравнения Пуассона : Subsystem
  Состояние БЛА : Outport
  wires:
  U1/1 -> Векторы ускорений действующих сил/1(U1)
  Bus Creator/1 -> Состояние БЛА/1
  Решение уравнения Пуассона/3(Psi) -> Векторы ускорений действующих сил/4(Psi), Bus Creator/9
  Решение уравнения Пуассона/1(Roll) -> Векторы ускорений действующих сил/3(Roll), Bus Creator/7
  Решение уравнения Пуассона/2(Pitch) -> Bus Creator/8, Векторы ускорений действующих сил/2(Pitch)
  Векторы ускорений действующих сил/1("Векторы ускорений, 3 x [3 x 1]") -> Bus Selector/1
  "Вектор ускорений, действующих сил"/1 -> Demux2/1, Demux/1
  Demux/1 -> Простр. движение Ц.М. БПЛА (Геогр. СК)/1(Acc X)  "AccX"
  Demux/2 -> Простр. движение Ц.М. БПЛА (Геогр. СК)/2(Acc Y)  "AccY"
  Demux/3 -> Простр. движение Ц.М. БПЛА (Геогр. СК)/3(AccZ)  "AccZ"
  Простр. движение Ц.М. БПЛА (Геогр. СК)/1("(X, Y, Z, phi, lambda)") -> Bus Selector2/1, Векторы ускорений действующих сил/6("(X, Y, Z, phi)")
  g/1 -> Векторы ускорений действующих сил/5(g)
  Demux2/1 -> Bus Creator/4  "AccX"
  Demux2/2 -> Bus Creator/5  "AccY"
  Demux2/3 -> Bus Creator/6  "AccZ"
  Простр. движение Ц.М. БПЛА (Геогр. СК)/3(Относительное и Кориолисово ускорение) -> Векторы ускорений действующих сил/7(Относительное и Кориолисово ускорение)
  Bus Selector/1 -> "Вектор ускорений, действующих сил"/1  "<Вектор ускорения силы тяги [3 x 1]>"
  Bus Selector/2 -> "Вектор ускорений, действующих сил"/2  "<Вектор Кориолисова ускорения [3 x 1]>"
  Bus Selector/3 -> "Вектор ускорений, действующих сил"/3  "<Вектор относительного ускорения [3 x 1]>"
  Bus Selector/4 -> "Вектор ускорений, действующих сил"/4  "<Вектор ускорения силы гравитации [3 x 1]>"
  Простр. движение Ц.М. БПЛА (Геогр. СК)/2((Vx,Vy,Vz)) -> Demux4/1
  Demux4/1 -> Bus Creator/13  "VelX"
  Demux4/2 -> Bus Creator/14  "VelY"
  Demux4/3 -> Bus Creator/15  "VelZ"
  Bus Selector2/1 -> Bus Creator/1, To Workspace1/1  "<X>"
  Bus Selector2/2 -> Bus Creator/2, To Workspace2/1  "<Y>"
  Bus Selector2/3 -> To Workspace3/1, Bus Creator/3  "<Z>"
  Bus Selector2/4 -> Bus Creator/16  "<phi>"
  Bus Selector2/5 -> Bus Creator/17  "<lambda>"
  "Север(0), Восток(0)"/1 -> Простр. движение Ц.М. БПЛА (Геогр. СК)/4("Север(0), Восток(0)")
  U2/1 -> Моменты управляемых сил/1(U2)
  U4/1 -> Моменты управляемых сил/2(U4)
  U3/1 -> Моменты управляемых сил/3(U3)
  Моменты управляемых сил/1("(Mx,My, Mz)") -> Demux1/1  "Управляемые, [3 x 1]"
  Demux1/1 -> Integrator/1
  Demux1/2 -> Integrator1/1
  Demux1/3 -> Integrator2/1
  Integrator/1 -> Mux/1
  Integrator1/1 -> Mux/2
  Integrator2/1 -> Mux/3
  Mux/1 -> Решение уравнения Пуассона/1(AngVelocity), Demux3/1
  Demux3/1 -> Bus Creator/10  "AngX"
  Demux3/2 -> Bus Creator/11  "AngY"
  Demux3/3 -> Bus Creator/12  "AngZ"

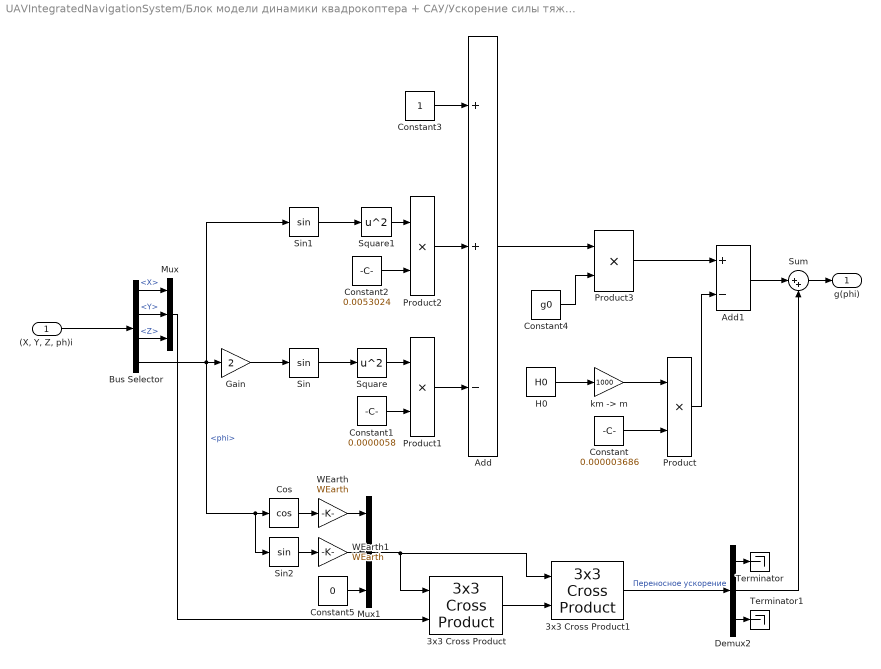
== system UAVIntegratedNavigationSystem/Блок модели динамики квадрокоптера + САУ/Ускорение силы тяжести на широте phi ==
  "(X, Y, Z, ph)i" : Inport
  3x3 Cross Product : sharedutil/3x3 Cross Product  aMode=aMode
      settings: SourceProductBaseCode=AE,PW,MT,UV,VE,VP
  3x3 Cross Product1 : sharedutil/3x3 Cross Product  aMode=aMode
      settings: SourceProductBaseCode=AE,PW,MT,UV,VE,VP
  Add : Sum  Inputs=++-
  Add1 : Sum  Inputs=+-
  Bus Selector : BusSelector  OutputSignals=X,Y,Z,phi
  Constant : Constant  Value=0.000003686
  Constant1 : Constant  Value=0.0000058
  Constant2 : Constant  Value=0.0053024
  Constant3 : Constant
  Constant4 : Constant  Value=g0
  Constant5 : Constant  Value=0
  Cos : Trigonometry  Operator=cos
  Demux2 : Demux  Outputs=3
  Gain : Gain  Gain=2
  H0 : Constant  Value=H0
  Mux : Mux  Inputs=3
  Mux1 : Mux  Inputs=3
  Product{,1..3} (4 alike) : Product
  Sin : Trigonometry
  Sin1 : Trigonometry
  Sin2 : Trigonometry
  Square : Math  Operator=square  SaturateOnIntegerOverflow=on
  Square1 : Math  Operator=square  SaturateOnIntegerOverflow=on
  Sum : Sum  Inputs=|++
  Terminator : Terminator
  Terminator1 : Terminator
  WEarth : Gain  Gain=WEarth
  WEarth1 : Gain  Gain=WEarth
  "km -> m" : Gain  Gain=1000
  g(phi) : Outport
  wires:
  H0/1 -> "km -> m"/1
  "km -> m"/1 -> Product/1
  Constant/1 -> Product/2
  Gain/1 -> Sin/1
  Sin/1 -> Square/1
  Square/1 -> Product1/1
  Constant1/1 -> Product1/2
  Sin1/1 -> Square1/1
  Constant2/1 -> Product2/2
  Square1/1 -> Product2/1
  Product1/1 -> Add/3
  Product2/1 -> Add/2
  Constant3/1 -> Add/1
  Add/1 -> Product3/1
  Constant4/1 -> Product3/2
  Product3/1 -> Add1/1
  Product/1 -> Add1/2
  Add1/1 -> Sum/1
  Bus Selector/4 -> Sin1/1, Gain/1, Sin2/1, Cos/1  "<phi>"
  3x3 Cross Product1/1 -> Demux2/1  "Переносное ускорение"
  Mux1/1 -> 3x3 Cross Product1/1, 3x3 Cross Product/1
  Sin2/1 -> WEarth1/1
  3x3 Cross Product/1 -> 3x3 Cross Product1/2
  WEarth1/1 -> Mux1/2
  Mux/1 -> 3x3 Cross Product/2
  Constant5/1 -> Mux1/3
  Demux2/1 -> Terminator/1
  Demux2/3 -> Terminator1/1
  WEarth/1 -> Mux1/1
  Cos/1 -> WEarth/1
  "(X, Y, Z, ph)i"/1 -> Bus Selector/1
  Bus Selector/1 -> Mux/1  "<X>"
  Bus Selector/2 -> Mux/2  "<Y>"
  Bus Selector/3 -> Mux/3  "<Z>"
  Demux2/2 -> Sum/2
  Sum/1 -> g(phi)/1

== system UAVIntegratedNavigationSystem/Блок создания траектории движения БЛА/If Action Subsystem ==
  XZ(0) : Inport
  t : Inport  Port=2
  TAltitude : Inport  Port=3
  Action Port : ActionPort  ActionPortLabel=if(u1 <= u2)
  Demux : Demux  Outputs=2
  Mux : Mux  Inputs=2
  Start Path Coordinate : MATLAB Function  TreatAsAtomicUnit=on
  Out1 : Outport
  wires:
  TAltitude/1 -> Start Path Coordinate/2(TAltitude)
  Start Path Coordinate/1(X) -> Mux/1
  Start Path Coordinate/2(Z) -> Mux/2
  Mux/1 -> Out1/1
  Demux/1 -> Start Path Coordinate/3(NorthInit)
  XZ(0)/1 -> Demux/1
  Demux/2 -> Start Path Coordinate/4(EastInit)
  t/1 -> Start Path Coordinate/1(t)

== system UAVIntegratedNavigationSystem/Блок создания траектории движения БЛА/If Action Subsystem1 ==
  XZ : Inport
  Action Port : ActionPort  ActionPortLabel=else
  Out1 : Outport
  wires:
  XZ/1 -> Out1/1

== system UAVIntegratedNavigationSystem/Блок создания траектории движения БЛА/If Action Subsystem2 ==
  In1 : Inport
  Action Port : ActionPort  ActionPortLabel=if(u1 > u2)
  Out1 : Outport
  wires:
  In1/1 -> Out1/1

== system UAVIntegratedNavigationSystem/Блок создания траектории движения БЛА/If Action Subsystem3 ==
  Action Port : ActionPort  ActionPortLabel=else
  Constant : Constant  Value=0
  Out1 : Outport
  wires:
  Constant/1 -> Out1/1

== system UAVIntegratedNavigationSystem/Блок создания траектории движения БЛА/Выбор траектории движения БЛА ==
  t : Inport
  TAltitude : Inport  Port=2
  Constant : Constant  Value=2
  Eight Path : MATLAB Function  TreatAsAtomicUnit=on
  Line Path : MATLAB Function  TreatAsAtomicUnit=on
  Multiport Switch : MultiPortSwitch
  Multiport Switch1 : MultiPortSwitch
  Mux{1..6} (6 alike) : Mux  Inputs=2
  Slider : SliderBlock  ScaleMin=1  ScaleMax=3  TickInterval=1
  Snake Path : MATLAB Function  TreatAsAtomicUnit=on
  X(0) : Constant  Value=0
  X(0)1 : Constant  Value=1000
  XZ : Outport
  XZ(0) : Outport  Port=2
  wires:
  Eight Path/1(X) -> Mux4/1  "X заданная"
  t/1 -> Snake Path/1(t), Eight Path/1(t), Line Path/1(t)
  Snake Path/2(Z) -> Mux5/2  "Z  заданная"
  Eight Path/2(Z) -> Mux4/2  "Z  заданная"
  Mux2/1 -> Multiport Switch/2
  Snake Path/1(X) -> Mux5/1  "X заданная"
  Mux5/1 -> Multiport Switch/4
  Line Path/1(X) -> Mux2/1  "X заданная"
  Mux4/1 -> Multiport Switch/3
  Constant/1 -> Multiport Switch/1, Multiport Switch1/1
  Line Path/2(Z) -> Mux2/2  "Z  заданная"
  Multiport Switch/1 -> XZ/1
  Mux1/1 -> Multiport Switch1/2
  Mux3/1 -> Multiport Switch1/3
  X(0)/1 -> Mux6/2, Mux6/1, Mux3/2, Mux1/2, Mux1/1
  X(0)1/1 -> Eight Path/2(NorthEight), Mux3/1
  Mux6/1 -> Multiport Switch1/4
  Multiport Switch1/1 -> XZ(0)/1
  TAltitude/1 -> Eight Path/3(TAltitude), Snake Path/2(TAltitude), Line Path/2(TAltitude)

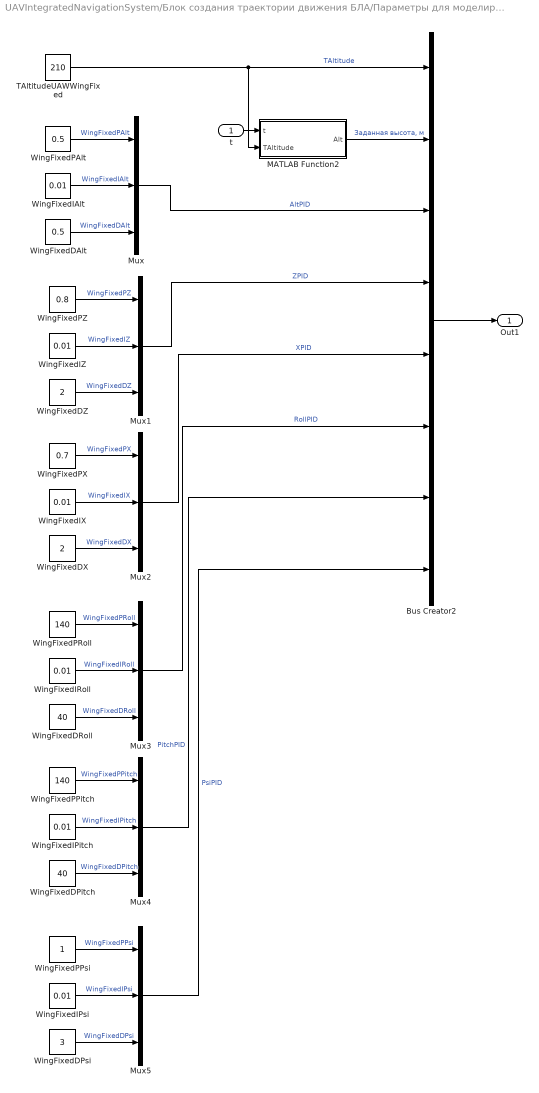
== system UAVIntegratedNavigationSystem/Блок создания траектории движения БЛА/Параметры для моделирования самолета типа 1 ==
  t : Inport
  Bus Creator2 : BusCreator  Inputs=8
  MATLAB Function2 : MATLAB Function  TreatAsAtomicUnit=on
  Mux{,1..5} (6 alike) : Mux  Inputs=3
  TAltitudeUAWWingFixed : Constant  Value=210
  WingFixedDAlt : Constant  Value=0.5
  WingFixedDPitch : Constant  Value=40
  WingFixedDPsi : Constant  Value=3
  WingFixedDRoll : Constant  Value=40
  WingFixedDX : Constant  Value=2
  WingFixedDZ : Constant  Value=2
  WingFixedIAlt : Constant  Value=0.01
  WingFixedIPitch : Constant  Value=0.01
  WingFixedIPsi : Constant  Value=0.01
  WingFixedIRoll : Constant  Value=0.01
  WingFixedIX : Constant  Value=0.01
  WingFixedIZ : Constant  Value=0.01
  WingFixedPAlt : Constant  Value=0.5
  WingFixedPPitch : Constant  Value=140
  WingFixedPPsi : Constant
  WingFixedPRoll : Constant  Value=140
  WingFixedPX : Constant  Value=0.7
  WingFixedPZ : Constant  Value=0.8
  Out1 : Outport
  wires:
  MATLAB Function2/1(Alt) -> Bus Creator2/2  "Заданная высота, м"
  t/1 -> MATLAB Function2/1(t)
  Bus Creator2/1 -> Out1/1
  TAltitudeUAWWingFixed/1 -> MATLAB Function2/2(TAltitude), Bus Creator2/1  "TAltitude"
  WingFixedDAlt/1 -> Mux/3  "WingFixedDAlt"
  WingFixedPZ/1 -> Mux1/1  "WingFixedPZ"
  WingFixedIZ/1 -> Mux1/2  "WingFixedIZ"
  WingFixedDZ/1 -> Mux1/3  "WingFixedDZ"
  WingFixedPX/1 -> Mux2/1  "WingFixedPX"
  WingFixedDX/1 -> Mux2/3  "WingFixedDX"
  WingFixedIAlt/1 -> Mux/2  "WingFixedIAlt"
  WingFixedIX/1 -> Mux2/2  "WingFixedIX"
  WingFixedPAlt/1 -> Mux/1  "WingFixedPAlt"
  Mux/1 -> Bus Creator2/3  "AltPID"
  Mux1/1 -> Bus Creator2/4  "ZPID"
  Mux2/1 -> Bus Creator2/5  "XPID"
  Mux3/1 -> Bus Creator2/6  "RollPID"
  WingFixedPPsi/1 -> Mux5/1  "WingFixedPPsi"
  Mux4/1 -> Bus Creator2/7  "PitchPID"
  WingFixedDPsi/1 -> Mux5/3  "WingFixedDPsi"
  WingFixedIPsi/1 -> Mux5/2  "WingFixedIPsi"
  WingFixedIPitch/1 -> Mux4/2  "WingFixedIPitch"
  WingFixedDPitch/1 -> Mux4/3  "WingFixedDPitch"
  Mux5/1 -> Bus Creator2/8  "PsiPID"
  WingFixedPRoll/1 -> Mux3/1  "WingFixedPRoll"
  WingFixedDRoll/1 -> Mux3/3  "WingFixedDRoll"
  WingFixedIRoll/1 -> Mux3/2  "WingFixedIRoll"
  WingFixedPPitch/1 -> Mux4/1  "WingFixedPPitch"

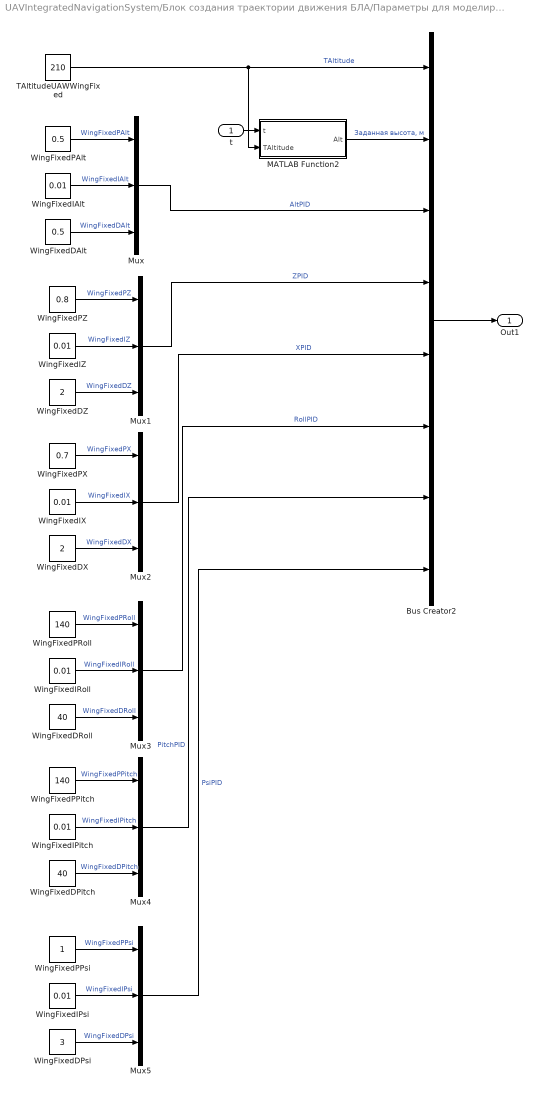
== system UAVIntegratedNavigationSystem/Блок создания траектории движения БЛА/Параметры для моделирования самолета типа 2 ==
  t : Inport
  Bus Creator2 : BusCreator  Inputs=8
  MATLAB Function2 : MATLAB Function  TreatAsAtomicUnit=on
  Mux{,1..5} (6 alike) : Mux  Inputs=3
  TAltitudeUAWWingFixed : Constant  Value=210
  WingFixedDAlt : Constant  Value=0.5
  WingFixedDPitch : Constant  Value=40
  WingFixedDPsi : Constant  Value=3
  WingFixedDRoll : Constant  Value=40
  WingFixedDX : Constant  Value=2
  WingFixedDZ : Constant  Value=2
  WingFixedIAlt : Constant  Value=0.01
  WingFixedIPitch : Constant  Value=0.01
  WingFixedIPsi : Constant  Value=0.01
  WingFixedIRoll : Constant  Value=0.01
  WingFixedIX : Constant  Value=0.01
  WingFixedIZ : Constant  Value=0.01
  WingFixedPAlt : Constant  Value=0.5
  WingFixedPPitch : Constant  Value=140
  WingFixedPPsi : Constant
  WingFixedPRoll : Constant  Value=140
  WingFixedPX : Constant  Value=0.7
  WingFixedPZ : Constant  Value=0.8
  Out1 : Outport
  wires:
  MATLAB Function2/1(Alt) -> Bus Creator2/2  "Заданная высота, м"
  t/1 -> MATLAB Function2/1(t)
  Bus Creator2/1 -> Out1/1
  TAltitudeUAWWingFixed/1 -> MATLAB Function2/2(TAltitude), Bus Creator2/1  "TAltitude"
  WingFixedDAlt/1 -> Mux/3  "WingFixedDAlt"
  WingFixedPZ/1 -> Mux1/1  "WingFixedPZ"
  WingFixedIZ/1 -> Mux1/2  "WingFixedIZ"
  WingFixedDZ/1 -> Mux1/3  "WingFixedDZ"
  WingFixedPX/1 -> Mux2/1  "WingFixedPX"
  WingFixedDX/1 -> Mux2/3  "WingFixedDX"
  WingFixedIAlt/1 -> Mux/2  "WingFixedIAlt"
  WingFixedIX/1 -> Mux2/2  "WingFixedIX"
  WingFixedPAlt/1 -> Mux/1  "WingFixedPAlt"
  Mux/1 -> Bus Creator2/3  "AltPID"
  Mux1/1 -> Bus Creator2/4  "ZPID"
  Mux2/1 -> Bus Creator2/5  "XPID"
  Mux3/1 -> Bus Creator2/6  "RollPID"
  WingFixedPPsi/1 -> Mux5/1  "WingFixedPPsi"
  Mux4/1 -> Bus Creator2/7  "PitchPID"
  WingFixedDPsi/1 -> Mux5/3  "WingFixedDPsi"
  WingFixedIPsi/1 -> Mux5/2  "WingFixedIPsi"
  WingFixedIPitch/1 -> Mux4/2  "WingFixedIPitch"
  WingFixedDPitch/1 -> Mux4/3  "WingFixedDPitch"
  Mux5/1 -> Bus Creator2/8  "PsiPID"
  WingFixedPRoll/1 -> Mux3/1  "WingFixedPRoll"
  WingFixedDRoll/1 -> Mux3/3  "WingFixedDRoll"
  WingFixedIRoll/1 -> Mux3/2  "WingFixedIRoll"
  WingFixedPPitch/1 -> Mux4/1  "WingFixedPPitch"

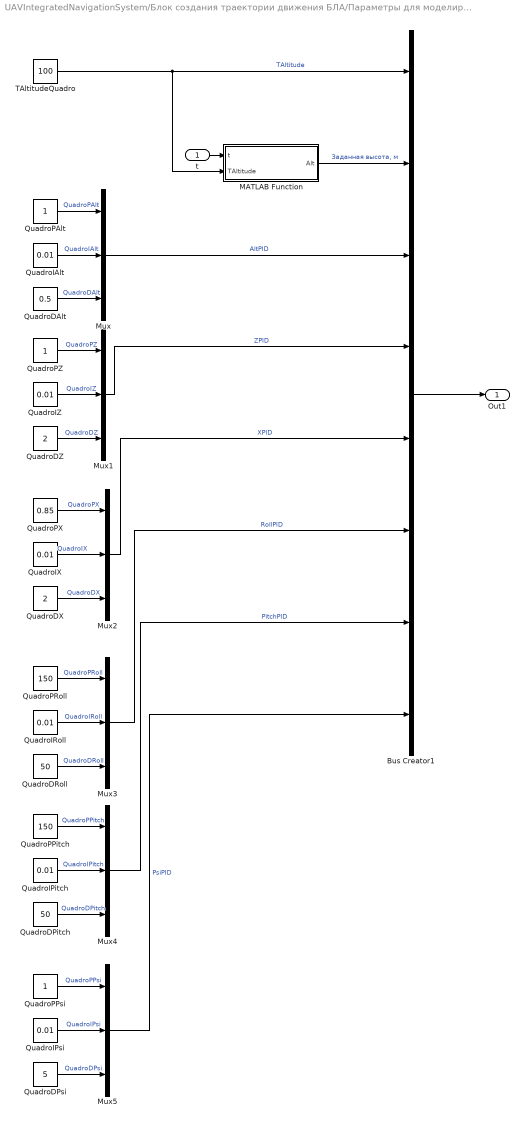
== system UAVIntegratedNavigationSystem/Блок создания траектории движения БЛА/Параметры для моделирования квадрокоптера ==
  t : Inport
  Bus Creator1 : BusCreator  Inputs=8
  MATLAB Function : MATLAB Function  TreatAsAtomicUnit=on
  Mux{,1..5} (6 alike) : Mux  Inputs=3
  QuadroDAlt : Constant  Value=0.5
  QuadroDPitch : Constant  Value=50
  QuadroDPsi : Constant  Value=5
  QuadroDRoll : Constant  Value=50
  QuadroDX : Constant  Value=2
  QuadroDZ : Constant  Value=2
  QuadroIAlt : Constant  Value=0.01
  QuadroIPitch : Constant  Value=0.01
  QuadroIPsi : Constant  Value=0.01
  QuadroIRoll : Constant  Value=0.01
  QuadroIX : Constant  Value=0.01
  QuadroIZ : Constant  Value=0.01
  QuadroPAlt : Constant
  QuadroPPitch : Constant  Value=150
  QuadroPPsi : Constant
  QuadroPRoll : Constant  Value=150
  QuadroPX : Constant  Value=0.85
  QuadroPZ : Constant
  TAltitudeQuadro : Constant  Value=100
  Out1 : Outport
  wires:
  TAltitudeQuadro/1 -> MATLAB Function/2(TAltitude), Bus Creator1/1  "TAltitude"
  MATLAB Function/1(Alt) -> Bus Creator1/2  "Заданная высота, м"
  Bus Creator1/1 -> Out1/1
  t/1 -> MATLAB Function/1(t)
  QuadroPAlt/1 -> Mux/1  "QuadroPAlt"
  QuadroDZ/1 -> Mux1/3  "QuadroDZ"
  QuadroIZ/1 -> Mux1/2  "QuadroIZ"
  QuadroPZ/1 -> Mux1/1  "QuadroPZ"
  QuadroIX/1 -> Mux2/2  "QuadroIX"
  QuadroDX/1 -> Mux2/3  "QuadroDX"
  QuadroPX/1 -> Mux2/1  "QuadroPX"
  Mux/1 -> Bus Creator1/3  "AltPID"
  QuadroIAlt/1 -> Mux/2  "QuadroIAlt"
  QuadroDAlt/1 -> Mux/3  "QuadroDAlt"
  Mux1/1 -> Bus Creator1/4  "ZPID"
  Mux2/1 -> Bus Creator1/5  "XPID"
  QuadroPRoll/1 -> Mux3/1  "QuadroPRoll"
  QuadroIRoll/1 -> Mux3/2  "QuadroIRoll"
  QuadroDRoll/1 -> Mux3/3  "QuadroDRoll"
  Mux3/1 -> Bus Creator1/6  "RollPID"
  QuadroDPitch/1 -> Mux4/3  "QuadroDPitch"
  QuadroIPitch/1 -> Mux4/2  "QuadroIPitch"
  Mux4/1 -> Bus Creator1/7  "PitchPID"
  QuadroPPitch/1 -> Mux4/1  "QuadroPPitch"
  Mux5/1 -> Bus Creator1/8  "PsiPID"
  QuadroPPsi/1 -> Mux5/1  "QuadroPPsi"
  QuadroIPsi/1 -> Mux5/2  "QuadroIPsi"
  QuadroDPsi/1 -> Mux5/3  "QuadroDPsi"

== system UAVIntegratedNavigationSystem/Моделирование задержки при переключении режимов работы КОИ/If Action Subsystem ==
  In1 : Inport
  Action Port : ActionPort  ActionPortLabel=if(u1 ~= 0)
  Out1 : Outport
  wires:
  In1/1 -> Out1/1

== system UAVIntegratedNavigationSystem/Моделирование задержки при переключении режимов работы КОИ/If Action Subsystem1 ==
  Индекс режима КОИ : Inport
  Action Port : ActionPort  ActionPortLabel=else
  Out1 : Outport
  wires:
  Индекс режима КОИ/1 -> Out1/1

== system UAVIntegratedNavigationSystem/Моделирование задержки при переключении режимов работы КОИ/If Action Subsystem2 ==
  In1 : Inport
  Action Port : ActionPort  ActionPortLabel=if(u1 > delay)
  Out1 : Outport
  wires:
  In1/1 -> Out1/1

== system UAVIntegratedNavigationSystem/Моделирование задержки при переключении режимов работы КОИ/If Action Subsystem3 ==
  KOI : Inport
  Action Port : ActionPort  ActionPortLabel=else
  Out1 : Outport
  wires:
  KOI/1 -> Out1/1

== system UAVIntegratedNavigationSystem/Показания АИОН + ЛД/Измерения АИОН + ЛД ==
  "Состояние БЛА " : Inport
  Add : Sum
  Add1 : Sum
  Bus Creator : BusCreator  Inputs=3
  Bus Selector : BusSelector  OutputSignals=X,Y,Z
  Demux : Demux  Outputs=2
  Mux1 : Mux  Inputs=2
  Вектор случайных аддитивных ошибок в определении высоты местоположения БЛА : Subsystem
  Вектор случайных аддитивных ошибок в определении координат местоположения БЛА : Subsystem
  "Измерения АИОН + ЛД,  [3 x 1]" : Outport
  wires:
  Mux1/1 -> Add/2
  "Состояние БЛА "/1 -> Bus Selector/1
  Вектор случайных аддитивных ошибок в определении высоты местоположения БЛА/1(Вектор измерительных шумов [1x1]) -> Add1/2
  Bus Creator/1 -> "Измерения АИОН + ЛД,  [3 x 1]"/1
  Вектор случайных аддитивных ошибок в определении координат местоположения БЛА/1(Вектор измерительных шумов [2x1]) -> Add/1
  Bus Selector/3 -> Mux1/2  "<Z>"
  Bus Selector/1 -> Mux1/1  "<X>"
  Bus Selector/2 -> Add1/1  "<Y>"
  Add/1 -> Demux/1  "Вектор координат по АИОН, [2 x 1]"
  Add1/1 -> Bus Creator/2  "Altitude_AION"
  Demux/1 -> Bus Creator/1  "X_Geo_AION"
  Demux/2 -> Bus Creator/3  "Z_Geo_AION"

== system UAVIntegratedNavigationSystem/Показания приемника ГНСС/Измерения ГНСС ==
  "Состояние БЛА " : Inport
  Add : Sum
  Add1 : Sum
  Add2 : Sum
  Bus Creator : BusCreator  Inputs=3
  Bus Selector : BusSelector  OutputSignals=X,Y,Z,VelX,VelY,VelZ,Roll,Pitch,Psi
  Mux1 : Mux  Inputs=3
  Mux2 : Mux  Inputs=3
  Mux3 : Mux  Inputs=3
  Вектор случайных аддитивных ошибок в определении координат местопложения БЛА : Subsystem
  Вектор случайных аддитивных ошибок в определении ориентации БЛА : Subsystem
  Вектор случайных аддитивных ошибок в определении проекций скорости  БЛА : Subsystem
  "Измерения приемника ГНСС, 2 x [3 x 1]" : Outport
  wires:
  Bus Selector/2 -> Mux1/2  "<Y>"
  Mux1/1 -> Add/2
  "Состояние БЛА "/1 -> Bus Selector/1
  Mux2/1 -> Add1/1
  Bus Selector/5 -> Mux2/2  "<VelY>"
  Bus Selector/6 -> Mux2/3  "<VelZ>"
  Bus Selector/4 -> Mux2/1  "<VelX>"
  Вектор случайных аддитивных ошибок в определении проекций скорости  БЛА/1(Вектор измерительных шумов [3x1]) -> Add1/2
  Bus Creator/1 -> "Измерения приемника ГНСС, 2 x [3 x 1]"/1
  Add/1 -> Bus Creator/1  "Вектор координат по ГНСС, [3 x 1]"
  Add1/1 -> Bus Creator/2  "Вектор проекций скоростей по ГНСС, [3 x 1]"
  Вектор случайных аддитивных ошибок в определении координат местопложения БЛА/1(Вектор измерительных шумов [3x1]) -> Add/1
  Bus Selector/3 -> Mux1/3  "<Z>"
  Bus Selector/1 -> Mux1/1  "<X>"
  Add2/1 -> Bus Creator/3  "Вектор углов по ГНСС, [3 x 1]"
  Bus Selector/7 -> Mux3/1  "<Roll>"
  Mux3/1 -> Add2/1
  Вектор случайных аддитивных ошибок в определении ориентации БЛА/1(Вектор измерительных шумов [3x1]) -> Add2/2
  Bus Selector/9 -> Mux3/2  "<Psi>"
  Bus Selector/8 -> Mux3/3  "<Pitch>"

== system UAVIntegratedNavigationSystem/Subsystem1/Функционирование АИОН/If Action Subsystem1 ==
  In1 : Inport
  Action Port : ActionPort  ActionPortLabel=if(u1 == 2)
  Out1 : Outport
  wires:
  In1/1 -> Out1/1

== system UAVIntegratedNavigationSystem/Subsystem1/Функционирование АИОН/If Action Subsystem3 ==
  Action Port : ActionPort  ActionPortLabel=else
  Constant : Constant  Value=-1
  Out1 : Outport
  wires:
  Constant/1 -> Out1/1

== system UAVIntegratedNavigationSystem/Subsystem1/Функционирование АИОН/If Action Subsystem4 ==
  Action Port : ActionPort  ActionPortLabel=if(u1 == -1)
  Bus Creator : BusCreator  Inputs=3
  NaN : Constant  Value=NaN  OutDataTypeStr=Inherit: Inherit via back propagation
  NaN1 : Constant  Value=NaN  OutDataTypeStr=Inherit: Inherit via back propagation
  NaN2 : Constant  Value=NaN  OutDataTypeStr=Inherit: Inherit via back propagation
  Out1 : Outport
  wires:
  NaN/1 -> Bus Creator/1
  NaN1/1 -> Bus Creator/2
  NaN2/1 -> Bus Creator/3
  Bus Creator/1 -> Out1/1

== system UAVIntegratedNavigationSystem/Subsystem1/Функционирование АИОН/If Action Subsystem5 ==
  In1 : Inport
  Action Port : ActionPort  ActionPortLabel=else
  Out1 : Outport
  wires:
  In1/1 -> Out1/1

== system UAVIntegratedNavigationSystem/Subsystem1/Функционирование приемника ГНСС/If Action Subsystem1 ==
  In1 : Inport
  Action Port : ActionPort  ActionPortLabel=if(u1 == 1)
  Out1 : Outport
  wires:
  In1/1 -> Out1/1

== system UAVIntegratedNavigationSystem/Subsystem1/Функционирование приемника ГНСС/If Action Subsystem3 ==
  Action Port : ActionPort  ActionPortLabel=else
  Constant : Constant  Value=-1
  Out1 : Outport
  wires:
  Constant/1 -> Out1/1
